simulink model "Ex10_2_3_SimulinkSolutionNeg10yplusft"  (R2023a)
settings: Solver=VariableStepAuto  StartTime=0.0  StopTime=3  RelTol=1e-3
settings Model: Creator=Norb  LastModifiedBy=Norb

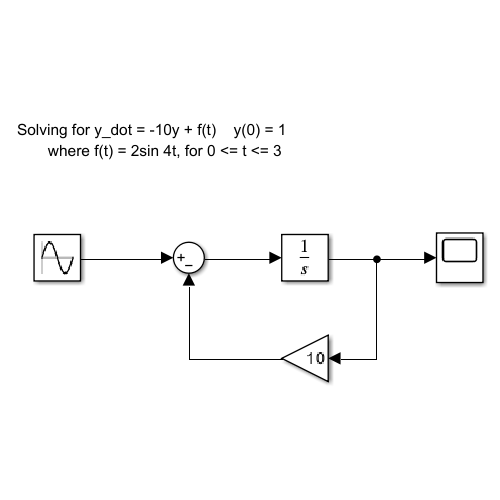
[thumbnail: Simulink's stored preview of the top-level diagram]
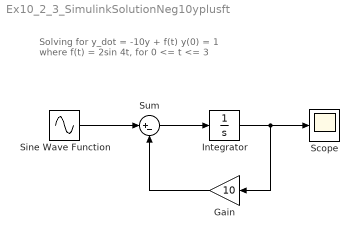
== system Ex10_2_3_SimulinkSolutionNeg10yplusft ==
  note: Solving for y_dot = -10y + f(t)	y(0) = 1
      | 	where f(t) = 2sin 4t, for 0 <= t <= 3
  Gain : Gain  Gain=10
  Integrator : Integrator
  Scope : Scope
  Sine Wave Function : Sin  SampleTime=0
  Sum : Sum  Inputs=|+-
  wires:
  Sine Wave Function/1 -> Sum/1
  Sum/1 -> Integrator/1
  Integrator/1 -> Gain/1, Scope/1
  Gain/1 -> Sum/2
